simulink model "lander_lqr"  (R2016b)
settings: Solver=VariableStepAuto  StartTime=0.0  StopTime=1000  RelTol=1e-3
values from neighbouring files (symbols this model uses):
  A = [O, I; N, O]    [main.m]
  B = [zeros(3,2); T]    [main.m]
  K = lqr(A,B,Q,R)    [main.m]
  r = [0 0 0 0 0 0]'    [main.m]
  x0 = [-20 20 0 0.1 2 0]'    [main.m]
undefined symbols (not defined in the file or in its folder): C, D
settings Model: Creator=elkman  LastModifiedBy=elkman

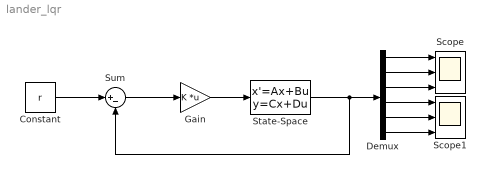
== system lander_lqr ==
  Constant : Constant  Value=r
  Demux : Demux  Outputs=6
  Gain : Gain  Gain=K  Multiplication=Matrix(K*u)
  Scope : Scope  NumInputPorts=3
  Scope1 : Scope  NumInputPorts=3
  State-Space : StateSpace  A=A  B=B  C=C  D=D  X0=x0
  Sum : Sum  Inputs=|+-
  wires:
  State-Space/1 -> Sum/2, Demux/1
  Constant/1 -> Sum/1
  Sum/1 -> Gain/1
  Gain/1 -> State-Space/1
  Demux/1 -> Scope/1
  Demux/2 -> Scope/2
  Demux/3 -> Scope/3
  Demux/4 -> Scope1/1
  Demux/5 -> Scope1/2
  Demux/6 -> Scope1/3
